simulink model "Sliding_Mode1"  (R2020b)
settings: Solver=VariableStepAuto  StartTime=0.0  StopTime=20  RelTol=1e-3
settings Model: Creator=zhiyao  LastModifiedBy=zhiyao

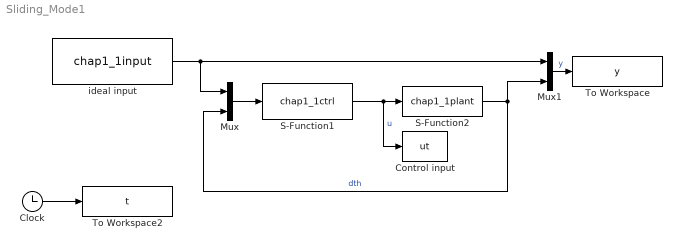
== system Sliding_Mode1 ==
  Clock : Clock
  Control input : ToWorkspace  VariableName=ut  SampleTime=-1
  Mux : Mux  Inputs=2
  Mux1 : Mux  Inputs=2
  S-Function1 : S-Function  FunctionName=chap1_1ctrl  SFunctionDeploymentMode=off  EnableBusSupport=off
  S-Function2 : S-Function  FunctionName=chap1_1plant  SFunctionDeploymentMode=off  EnableBusSupport=off
  To Workspace : ToWorkspace  VariableName=y  SampleTime=-1
  To Workspace2 : ToWorkspace  VariableName=t  SampleTime=-1
  ideal input : S-Function  FunctionName=chap1_1input  SFunctionDeploymentMode=off  EnableBusSupport=off
  wires:
  ideal input/1 -> Mux1/1, Mux/1
  S-Function1/1 -> Control input/1, S-Function2/1  "u"
  Mux/1 -> S-Function1/1
  Mux1/1 -> To Workspace/1  "y"
  S-Function2/1 -> Mux/2, Mux1/2  "dth"
  Clock/1 -> To Workspace2/1
